simulink model "Microgrid_w_BESS_Q4_1"  (R2024b)
settings: Solver=VariableStepAuto  StartTime=0.0  StopTime=4  RelTol=1e-3
undefined symbols (not defined in the file): DiscIntNeverNeededParam, ini_SoC, Ion, Lithium, Ts, Ts_Control
libraries: simulink x5, ee_lib x5, spsParallelRLCBranchLib x4, nesl_utility x4, spsCurrentVoltageSimscapeInterfaceLib x3, powerlib_extras x3, spsThreePhaseVIMeasurementLib x2, spsSeriesRLCBranchLib x2, spsMultimeterLib x2, spsThreePhaseSeriesRLCBranchLib x2, spsGroundLib x2, slpidlib x2
(part 2 of 2)

== matlab function Microgrid_w_BESS_Q4_1/BESS/BATT chg-dshg logic1/MATLAB Function5 ==
  data: Vdc input; D output; Vbatt input; I_batt_meas input; I_batt_ref_mag input; Ts input
function D = controller_discharging(Vdc, Vbatt, I_batt_meas, I_batt_ref_mag, Ts)
%#codegen
% Limits
Imax_discharge = -50;

% PI gains for discharging (tuned for stability and response)
Kp = 0.3; % Increased for faster error correction
Ki = 1; % Moderate integral action with anti-windup
Kd = 0.002; % Derivative term to dampen oscillations
persistent integral_error prev_error prev_I_batt_meas
if isempty(integral_error)
    integral_error = 0;
    prev_error = 0;
    prev_I_batt_meas = 0;
end

% Current reference
I_batt_ref = -I_batt_ref_mag; % Setpoint for discharging (e.g., -20A)

% Clamp current reference
I_batt_ref = max(I_batt_ref, Imax_discharge);

% PI control with derivative and anti-windup
error = I_batt_ref - I_batt_meas;
integral_error = max(min(integral_error + error * Ts, 200), -200); % Anti-windup clamp
derivative = (error - prev_error) / Ts - Kd * (I_batt_meas - prev_I_batt_meas) / Ts; % Damped derivative
PI_output = Kp * error + Ki * integral_error + derivative;
prev_error = error;
prev_I_batt_meas = I_batt_meas;

% Base duty calculation (boost mode)
D_base = 1 - Vbatt / Vdc;

% Total duty with adjusted limits
D = D_base + PI_output;
D = max(min(D, 0.55), 0.127); % New limits: 0.25 to 0.55

% Debugging
assignin('base', 'I_batt_ref', I_batt_ref);
assignin('base', 'I_batt_meas', I_batt_meas);
assignin('base', 'integral_error', integral_error);
assignin('base', 'D', D);
end

== matlab function Microgrid_w_BESS_Q4_1/BESS/BATT chg-dshg logic1/MATLAB Function6 ==
  data: Vdc input; D output; Vbatt input; I_batt_meas input; I_batt_ref_mag input; Ts input
function D = controller_charging(Vdc, Vbatt, I_batt_meas, I_batt_ref_mag, Ts)
%#codegen

% === Controller Parameters ===
Imax_charge = 50;
Kp_i = 2.0;           % Aggressive current loop gain
Ki_i = 20.0;          % Fast integral action
K_d  = 0.01;          % Optional derivative (lead) term

% === Persistent States ===
persistent integral_error_i prev_error_i I_batt_filt
if isempty(integral_error_i)
    integral_error_i = 0;
    prev_error_i = 0;
    I_batt_filt = I_batt_meas;
end

% === Filtered Current Measurement ===
alpha = 0.2;  % Faster response
I_batt_filt = alpha * I_batt_meas + (1 - alpha) * I_batt_filt;

% === Reference Current ===
I_batt_ref = min(I_batt_ref_mag, Imax_charge);  % Clamp ref

% === Skip Voltage Loop for Now ===
I_batt_ref_adj = I_batt_ref;

% === Inner Current Loop ===
error_i = I_batt_ref_adj - I_batt_filt;
d_error_i = (error_i - prev_error_i) / Ts;
prev_error_i = error_i;

PI_output_unsat = Kp_i * error_i + Ki_i * integral_error_i + K_d * d_error_i;

% === Disable Feedforward for Now ===
D_base = 0.5;

% === Saturate Duty and Apply Back-Calculation Anti-Windup ===
D_unsat = D_base + PI_output_unsat;
D_sat = max(min(D_unsat, 0.85), 0.127);
anti_windup_gain = 10;
integral_error_i = integral_error_i + Ts * (error_i + anti_windup_gain * (D_sat - D_unsat));

% === Final Duty Output ===
D = D_sat;

% === Debugging Outputs ===
assignin('base', 'I_batt_ref', I_batt_ref);
assignin('base', 'I_batt_ref_adj', I_batt_ref_adj);
assignin('base', 'I_batt_meas', I_batt_meas);
assignin('base', 'I_batt_filt', I_batt_filt);
assignin('base', 'error_i', error_i);
assignin('base', 'd_error_i', d_error_i);
assignin('base', 'integral_error_i', integral_error_i);
assignin('base', 'PI_output_unsat', PI_output_unsat);
assignin('base', 'D_base', D_base);
assignin('base', 'D_unsat', D_unsat);
assignin('base', 'D', D);
assignin('base', 'Vbatt', Vbatt);
assignin('base', 'Vdc', Vdc);
end
